simulink model "WTK_hybrid_random_1_staliro"  (R2021a)
settings: Solver=FixedStepAuto  StartTime=0.0  StopTime=T  FixedStep=Ts  RelTol=1e-3  EnableMultiTasking=on
InitFcn:
  | seed = randi(10000);
StartFcn:
  | seed = randi(10000);
undefined symbols (not defined in the file): DiscIntNeverNeededParam, isTerminate, Ts
libraries: simulink x3, rllib x2
settings Model: Creator=The MathWorks, Inc.  LastModifiedBy=ldy
settings SolverCC: AlgebraicLoopSolver=TrustRegion
settings DataIOCC: LimitDataPoints=on  SaveFormat=Array  ReturnWorkspaceOutputs=off
settings OptimizationCC: ExpressionDepthLimit=2147483647  InitFltsAndDblsToZero=on  LifeSpan=inf
settings DebuggingCC: SaveWithParameterizedLinksMsg=none  UnderspecifiedInitializationDetection=Classic  MergeDetectMultiDrivingBlocksExec=none  SignalResolutionControl=TryResolveAllWithWarning  MultiTaskDSMMsg=warning  FcnCallInpInsideContextMsg=warning  AllowSymbolicDim=off  StateNameClashWarn=warning  SFUnexpectedBacktrackingDiag=warning  SFNoUnconditionalDefaultTransitionDiag=warning  SFExecutionAtInitializationDiag=none  SFMachineParentedDataDiag=warning  ArithmeticOperatorsInVariantConditions=warning
settings HardwareCC: ProdBitPerPointer=32  ProdBitPerSizeT=32  ProdBitPerPtrDiffT=32  ProdLargestAtomicFloat=None  ProdIntDivRoundTo=Undefined  ProdEndianess=Unspecified  ProdWordSize=32  ProdHWDeviceType=Specified
settings ModelReferenceCC: PropagateSignalLabelsOutOfModel=off
settings SFSimCC: SimUseLocalCustomCode=off
settings RTWCC: RTWUseLocalCustomCode=off
settings CodeAppCC: StateflowObjectComments=on
settings GRTTargetCC: TargetFcnLib=ansi_tfl_tmw.mat  TargetLangStandard=C89/C90 (ANSI)  CombineOutputUpdateFcns=off  GRTInterface=on
settings ConfigComp: CovMetricSettings=dw  CovSaveCumulativeToWorkspaceVar=on  CovSaveSingleToWorkspaceVar=on  CovExternalEMLEnable=off

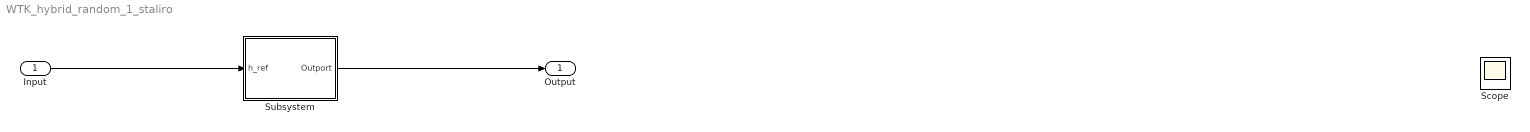
== system WTK_hybrid_random_1_staliro ==
  Input : Inport
  Subsystem : Subsystem
  Output : Outport
  Scope : Scope
  wires:
  Input/1 -> Subsystem/1(h_ref)
  Subsystem/1(Outport) -> Output/1

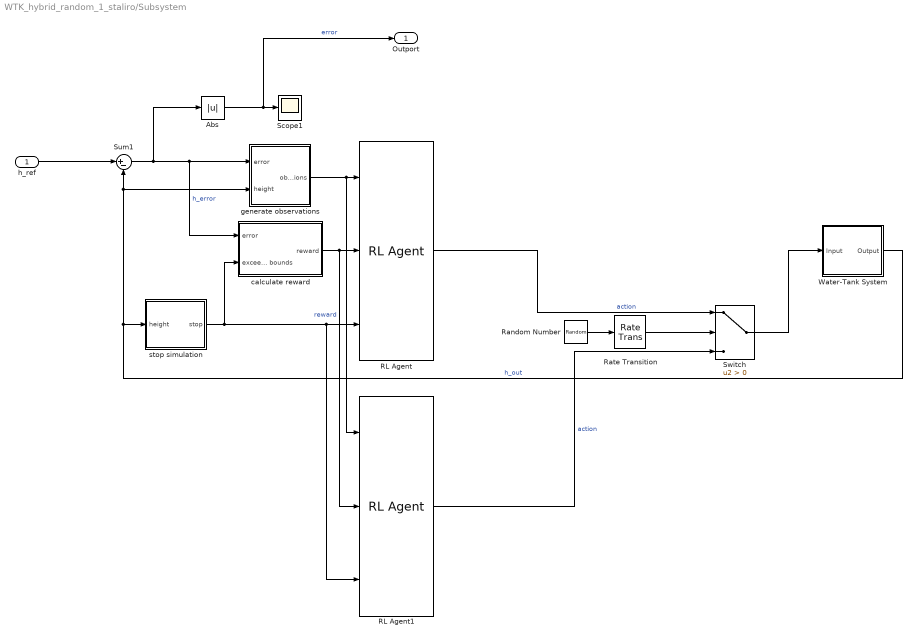
== system WTK_hybrid_random_1_staliro/Subsystem ==
  h_ref : Inport
  Abs : Abs
  RL Agent : rllib/RL Agent  Agent=agent  ExternalActionAsInput=off  ProvideCumRwd=off  TreatAsDirectFeedthrough=on
  RL Agent1 : rllib/RL Agent  Agent=agent_2  ExternalActionAsInput=off  ProvideCumRwd=off  TreatAsDirectFeedthrough=on
  Random Number : RandomNumber  Seed=seed  SampleTime=1
  Rate Transition : RateTransition  OutPortSampleTime=Ts
  Scope1 : Scope
  Sum1 : Sum  Inputs=|+-  SaturateOnIntegerOverflow=on
  Switch : Switch  Criteria=u2 > Threshold
  Water-Tank System : Subsystem
  calculate reward : Subsystem
  generate observations : Subsystem
  stop simulation : Subsystem
  Outport : Outport
  wires:
  Random Number/1 -> Rate Transition/1
  Switch/1 -> Water-Tank System/1(Input)
  stop simulation/1(stop) -> RL Agent1/3, RL Agent/3, calculate reward/2(exceeds bounds)
  generate observations/1(observations) -> RL Agent1/1, RL Agent/1
  Sum1/1 -> Abs/1, calculate reward/1(error), generate observations/1(error)  "h_error"
  calculate reward/1(reward) -> RL Agent1/2, RL Agent/2  "reward"
  Abs/1 -> Outport/1, Scope1/1  "error"
  h_ref/1 -> Sum1/1
  RL Agent1/1 -> Switch/3  "action"
  RL Agent/1 -> Switch/1  "action"
  Water-Tank System/1(Output) -> stop simulation/1(height), generate observations/2(height), Sum1/2  "h_out"
  Rate Transition/1 -> Switch/2

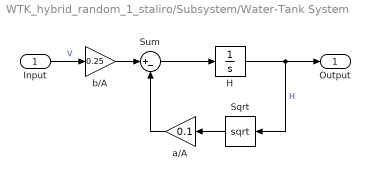
== system WTK_hybrid_random_1_staliro/Subsystem/Water-Tank System ==
  Input : Inport
  H : Integrator  InitialCondition=3  LimitOutput=on  LowerSaturationLimit=0
  Sqrt : Sqrt  OutputSignalType=real  SaturateOnIntegerOverflow=on
  Sum : Sum  Inputs=|+-  SaturateOnIntegerOverflow=on
  a/A : Gain  Gain=0.1  SaturateOnIntegerOverflow=on  OutDataTypeStr=Inherit: Same as input  ParamDataTypeStr=Inherit: Same as input
  b/A : Gain  Gain=0.25  SaturateOnIntegerOverflow=on  OutDataTypeStr=Inherit: Same as input  ParamDataTypeStr=Inherit: Same as input
  Output : Outport  VectorParamsAs1DForOutWhenUnconnected=off
  wires:
  b/A/1 -> Sum/1
  Sum/1 -> H/1
  H/1 -> Sqrt/1, Output/1  "H"
  Sqrt/1 -> a/A/1
  a/A/1 -> Sum/2
  Input/1 -> b/A/1  "V"

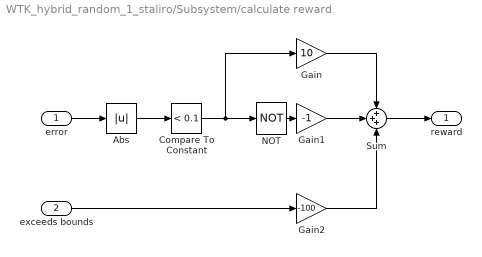
== system WTK_hybrid_random_1_staliro/Subsystem/calculate reward ==
  error : Inport
  exceeds bounds : Inport  Port=2
  Abs : Abs
  Compare To Constant : simulink/Logic and Bit Operations/Compare To Constant  relop=<  const=0.1  OutDataTypeStr=boolean
  Gain : Gain  Gain=10
  Gain1 : Gain  Gain=-1
  Gain2 : Gain  Gain=-100
  NOT : Logic  Operator=NOT  IconShape=distinctive  AllPortsSameDT=off  OutDataTypeStr=boolean
  Sum : Sum  Inputs=+++  OutDataTypeStr=double
  reward : Outport  VectorParamsAs1DForOutWhenUnconnected=off
  wires:
  Abs/1 -> Compare To Constant/1
  Gain2/1 -> Sum/3
  Gain/1 -> Sum/1
  Compare To Constant/1 -> NOT/1, Gain/1
  Gain1/1 -> Sum/2
  Sum/1 -> reward/1
  NOT/1 -> Gain1/1
  exceeds bounds/1 -> Gain2/1
  error/1 -> Abs/1

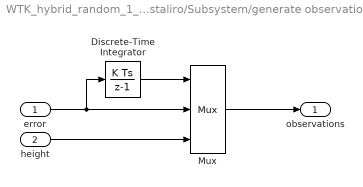
== system WTK_hybrid_random_1_staliro/Subsystem/generate observations ==
  error : Inport
  height : Inport  Port=2
  Discrete-Time Integrator : DiscreteIntegrator  SampleTime=Ts  ICPrevOutput=DiscIntNeverNeededParam  ICPrevScaledInput=DiscIntNeverNeededParam
  Mux : Mux  Inputs=3
  observations : Outport  VectorParamsAs1DForOutWhenUnconnected=off
  wires:
  height/1 -> Mux/3
  Discrete-Time Integrator/1 -> Mux/1
  error/1 -> Discrete-Time Integrator/1, Mux/2
  Mux/1 -> observations/1

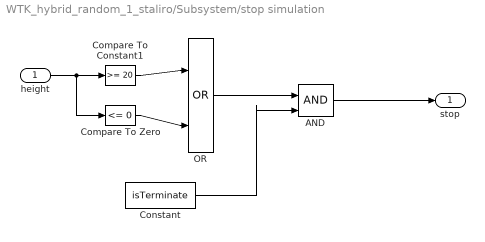
== system WTK_hybrid_random_1_staliro/Subsystem/stop simulation ==
  height : Inport
  AND : Logic  IconShape=distinctive  AllPortsSameDT=off  OutDataTypeStr=boolean
  Compare To Constant1 : simulink/Logic and Bit Operations/Compare To Constant  relop=>=  const=20  OutDataTypeStr=boolean
  Compare To Zero : simulink/Logic and Bit Operations/Compare To Zero  relop=<=  OutDataTypeStr=boolean
  Constant : Constant  Value=isTerminate
  OR : Logic  Operator=OR  IconShape=distinctive  AllPortsSameDT=off  OutDataTypeStr=boolean
  stop : Outport  VectorParamsAs1DForOutWhenUnconnected=off
  wires:
  height/1 -> Compare To Zero/1, Compare To Constant1/1
  Compare To Zero/1 -> OR/2
  Compare To Constant1/1 -> OR/1
  OR/1 -> AND/1
  AND/1 -> stop/1
  Constant/1 -> AND/2
